simulink model "Fuld_Model"  (R2016a)
settings: Solver=VariableStepAuto  StartTime=0.0  StopTime=5  RelTol=1e-3
values from neighbouring files (symbols this model uses):
  b = 0.000931    [Model.m]    (also in Projekt_disturbance.m; Rlocus.m = 3.5077e-06)
  J = 0.3    [Model.m]    (also in Projekt_disturbance.m = 0.00567; Rlocus.m = 3.2284e-06)
  K = 651/12    (= 54.25)    [Model.m]    (also in PID_test.m = 96.2958333333; Rlocus.m = 0.0274)
  Kb = 0.509    [Model.m]    (also in Projekt_disturbance.m)
  Km = 0.509    [Model.m]    (also in Projekt_disturbance.m)
  La = 0.0034    [Model.m]    (also in Projekt_disturbance.m)
  Ra = 7.101    [Model.m]    (also in Projekt_disturbance.m)
  T = 0.014    [Model.m]    (also in PID_test.m = 0.12)
libraries: simulink x1
settings Model: Creator=Kristian  LastModifiedBy=Kristian

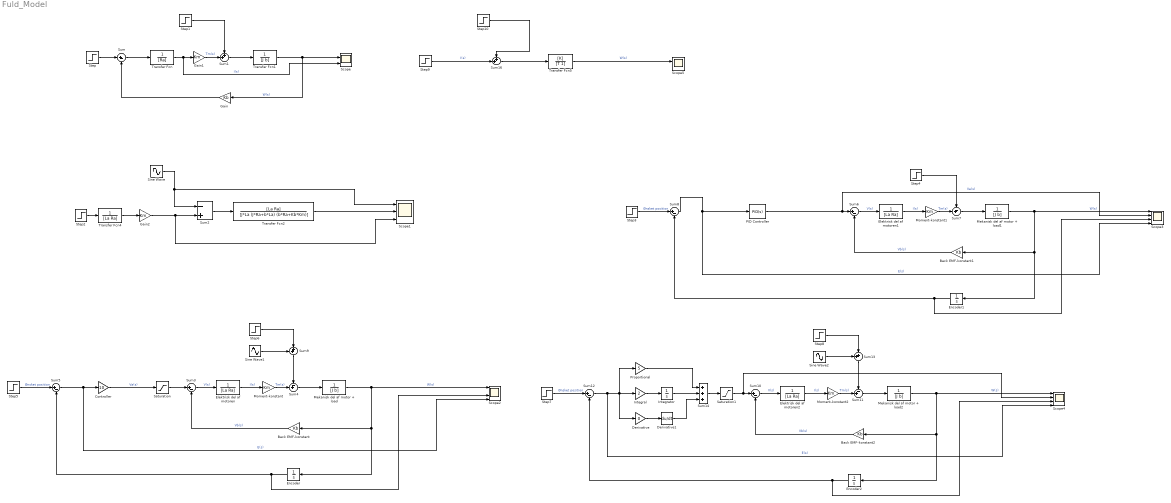
== system Fuld_Model ==
  Back EMF-konstant : Gain  Gain=Kb
  Back EMF-konstant1 : Gain  Gain=Kb
  Back EMF-konstant2 : Gain  Gain=Kb
  Controller : Gain  Gain=10  OutMin=-5  OutMax=5
  Derivative : Gain  Gain=0  OutMin=-5  OutMax=5
  Derivative1 : Derivative
  Elektrisk del af motoren : TransferFcn  Denominator=[La Ra]
  Elektrisk del af motoren1 : TransferFcn  Denominator=[La Ra]
  Elektrisk del af motoren2 : TransferFcn  Denominator=[La Ra]
  Encoder : Integrator
  Encoder1 : Integrator
  Encoder2 : Integrator
  Gain : Gain  Gain=Kb
  Gain1 : Gain  Gain=Km
  Gain2 : Gain  Gain=Km
  Integral : Gain  Gain=2  OutMin=-5  OutMax=5
  Integrator : Integrator
  Mekanisk del af motor + load : TransferFcn  Denominator=[J b]
  Mekanisk del af motor + load1 : TransferFcn  Denominator=[J b]
  Mekanisk del af motor + load2 : TransferFcn  Denominator=[J b]
  Moment-konstant : Gain  Gain=Km
  Moment-konstant1 : Gain  Gain=Km
  Moment-konstant2 : Gain  Gain=Km
  PID Controller : simulink/Continuous/PID Controller  Controller=PID  TimeDomain=Continuous-time  SampleTime=-1  IntegratorMethod=Forward Euler  FilterMethod=Forward Euler  Form=Parallel  UseFilter=on  ControllerParametersSource=internal  P=27.9731055534201  I=18.9419886143767  D=9.17860685589056  N=13264.9195073522  InitialConditionSource=internal  InitialConditionForIntegrator=0  InitialConditionForFilter=0  ExternalReset=none  LimitOutput=on  UpperSaturationLimit=5  LowerSaturationLimit=-5  LinearizeAsGain=on  AntiWindupMode=none  Kb=1  TrackingMode=off  Kt=1  PParamMin=[]  PParamMax=[]  IParamMin=[]  IParamMax=[]  DParamMin=[]  DParamMax=[]  NParamMin=[]  NParamMax=[]  KbParamMin=[]  KbParamMax=[]  KtParamMin=[]  KtParamMax=[]  POutMin=[]  POutMax=[]  IOutMin=[]  IOutMax=[]  DOutMin=[]  DOutMax=[]  NOutMin=[]  NOutMax=[]  KbOutMin=[]  KbOutMax=[]  KtOutMin=[]  KtOutMax=[]  IntegratorOutMin=[]  IntegratorOutMax=[]  FilterOutMin=[]  FilterOutMax=[]  SumOutMin=[]  SumOutMax=[]  SumI1OutMin=[]  SumI1OutMax=[]  SumI2OutMin=[]  SumI2OutMax=[]  SumI3OutMin=[]  SumI3OutMax=[]  SumDOutMin=[]  SumDOutMax=[]  SaturationOutMin=[]  SaturationOutMax=[]  IntegratorContinuousStateAttributes=''  IntegratorStateMustResolveToSignalObject=off  IntegratorRTWStateStorageClass=Auto  FilterContinuousStateAttributes=''  FilterStateMustResolveToSignalObject=off  FilterRTWStateStorageClass=Auto  DifferentiatorICPrevScaledInput=0  DifferentiatorOutMin=[]  DifferentiatorOutMax=[]
  Proportional : Gain  Gain=5  OutMin=-5  OutMax=5
  Saturation : Saturate  UpperLimit=5  LowerLimit=-5
  Saturation1 : Saturate  UpperLimit=5  LowerLimit=-5
  Scope : Scope  NumInputPorts=2
  Scope1 : Scope  NumInputPorts=3
  Scope2 : Scope  NumInputPorts=4
  Scope3 : Scope  NumInputPorts=4
  Scope4 : Scope  NumInputPorts=4
  Scope5 : Scope  NumInputPorts=2
  Sine Wave : Sin  Amplitude=0.3  Frequency=0.2  SampleTime=0
  Sine Wave1 : Sin  Amplitude=0  Frequency=0.1  SampleTime=0
  Sine Wave2 : Sin  Amplitude=0  Frequency=150  SampleTime=0
  Step : Step  After=12  SampleTime=0
  Step1 : Step  Time=10  After=0  SampleTime=0
  Step10 : Step  Time=10  After=0  SampleTime=0
  Step2 : Step  After=10  SampleTime=0
  Step3 : Step  After=10  SampleTime=0
  Step4 : Step  Time=10  After=0.3  SampleTime=0
  Step5 : Step  After=0  SampleTime=0
  Step6 : Step  Time=10  After=0.3  SampleTime=0
  Step7 : Step  After=10  SampleTime=0
  Step8 : Step  Time=10  After=0  SampleTime=0
  Step9 : Step  After=12  SampleTime=0
  Sum{,3,5..6,8,10,12} (7 alike) : Sum  Inputs=|+-
  Sum{1,9,13,16} (4 alike) : Sum  Inputs=++|
  Sum11 : Sum  Inputs=-+|
  Sum14 : Sum  Inputs=+++
  Sum2 : Sum  Inputs=-+
  Sum4 : Sum  Inputs=-+|
  Sum7 : Sum  Inputs=-+|
  Transfer Fcn : TransferFcn  Denominator=[Ra]
  Transfer Fcn1 : TransferFcn  Denominator=[J b]
  Transfer Fcn2 : TransferFcn  Numerator=[La Ra]  Denominator=[J*La (J*Ra+b*La) (b*Ra+Kb*Km)]
  Transfer Fcn4 : TransferFcn  Denominator=[La Ra]
  Transfer Fcn5 : TransferFcn  Numerator=[K]  Denominator=[T 1]
  wires:
  Sum/1 -> Transfer Fcn/1
  Gain/1 -> Sum/2
  Sum1/1 -> Transfer Fcn1/1
  Transfer Fcn1/1 -> Scope/1, Gain/1  "W(s)"
  Step1/1 -> Sum1/1
  Step/1 -> Sum/1
  Transfer Fcn/1 -> Scope/2, Gain1/1  "I(s)"
  Gain1/1 -> Sum1/2  "Tm(s)"
  Sum2/1 -> Transfer Fcn2/1
  Sine Wave/1 -> Scope1/1, Sum2/1
  Transfer Fcn2/1 -> Scope1/2
  Step2/1 -> Transfer Fcn4/1
  Gain2/1 -> Scope1/3, Sum2/2
  Transfer Fcn4/1 -> Gain2/1
  Sum3/1 -> Elektrisk del af motoren/1  "V(s)"
  Back EMF-konstant/1 -> Sum3/2  "Vb(s)"
  Sum4/1 -> Mekanisk del af motor + load/1
  Mekanisk del af motor + load/1 -> Scope2/1, Encoder/1, Back EMF-konstant/1  "W(s)"
  Controller/1 -> Saturation/1  "Va(s)"
  Elektrisk del af motoren/1 -> Moment-konstant/1  "I(s)"
  Moment-konstant/1 -> Sum4/2  "Tm(s)"
  Encoder/1 -> Scope2/3, Sum5/2
  Sum5/1 -> Scope2/4, Controller/1  "E(s)"
  Step5/1 -> Sum5/1  "Ønsket position"
  Saturation/1 -> Sum3/1
  Sum6/1 -> Elektrisk del af motoren1/1  "V(s)"
  Back EMF-konstant1/1 -> Sum6/2  "Vb(s)"
  Sum7/1 -> Mekanisk del af motor + load1/1
  Mekanisk del af motor + load1/1 -> Scope3/1, Encoder1/1, Back EMF-konstant1/1  "W(s)"
  Step4/1 -> Sum7/1
  PID Controller/1 -> Scope3/2, Sum6/1  "Va(s)"
  Elektrisk del af motoren1/1 -> Moment-konstant1/1  "I(s)"
  Moment-konstant1/1 -> Sum7/2  "Tm(s)"
  Encoder1/1 -> Scope3/3, Sum8/2
  Sum8/1 -> PID Controller/1, Scope3/4  "E(s)"
  Step3/1 -> Sum8/1  "Ønsket position"
  Step6/1 -> Sum9/2
  Sine Wave1/1 -> Sum9/1
  Sum9/1 -> Sum4/1
  Sum10/1 -> Elektrisk del af motoren2/1  "V(s)"
  Back EMF-konstant2/1 -> Sum10/2  "Vb(s)"
  Sum11/1 -> Mekanisk del af motor + load2/1
  Mekanisk del af motor + load2/1 -> Scope4/1, Encoder2/1, Back EMF-konstant2/1  "W(s)"
  Elektrisk del af motoren2/1 -> Moment-konstant2/1  "I(s)"
  Moment-konstant2/1 -> Sum11/2  "Tm(s)"
  Encoder2/1 -> Scope4/3, Sum12/2
  Sum12/1 -> Derivative/1, Integral/1, Proportional/1, Scope4/4  "E(s)"
  Step7/1 -> Sum12/1  "Ønsket position"
  Saturation1/1 -> Scope4/2, Sum10/1
  Step8/1 -> Sum13/2
  Sine Wave2/1 -> Sum13/1
  Sum13/1 -> Sum11/1
  Proportional/1 -> Sum14/1
  Sum14/1 -> Saturation1/1
  Integral/1 -> Integrator/1
  Integrator/1 -> Sum14/2
  Derivative/1 -> Derivative1/1
  Derivative1/1 -> Sum14/3
  Sum16/1 -> Transfer Fcn5/1
  Transfer Fcn5/1 -> Scope5/1  "W(s)"
  Step10/1 -> Sum16/1
  Step9/1 -> Sum16/2  "I(s)"
